simulink model "temp"  (R2015a)
settings: Solver=ode45  StartTime=0.0  StopTime=30.0  RelTol=1e-3
values from neighbouring files (symbols this model uses):
  Kyaw = 4*Kpsi*Km/Izz    (= 8.61428571429)    [Parametros.m]
  ty = 0.0002251891410    (= 0.000225189141)    [Parametros.m]
libraries: simulink x1
settings Model: Creator=DELL  LastModifiedBy=DELL

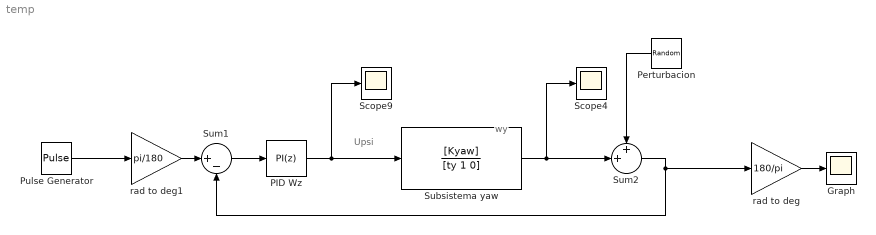
== system temp ==
  note: wy
  note: Upsi
  Graph : Scope
      settings: SaveName=ScopeData3
  PID Wz : simulink/Continuous/PID Controller  Controller=PI  TimeDomain=Discrete-time  SampleTime=0.01  IntegratorMethod=Forward Euler  FilterMethod=Forward Euler  Form=Ideal  UseFilter=on  ControllerParametersSource=internal  P=2.01  I=0.142  D=0.0957187049121133  N=189.58120119176  InitialConditionSource=internal  InitialConditionForIntegrator=0  InitialConditionForFilter=0  ExternalReset=none  LimitOutput=on  UpperSaturationLimit=1  LowerSaturationLimit=-1  LinearizeAsGain=on  AntiWindupMode=back-calculation  Kb=0.1  TrackingMode=off  Kt=1  PParamMin=[]  PParamMax=[]  IParamMin=[]  IParamMax=[]  DParamMin=[]  DParamMax=[]  NParamMin=[]  NParamMax=[]  KbParamMin=[]  KbParamMax=[]  KtParamMin=[]  KtParamMax=[]  POutMin=[]  POutMax=[]  IOutMin=[]  IOutMax=[]  DOutMin=[]  DOutMax=[]  NOutMin=[]  NOutMax=[]  KbOutMin=[]  KbOutMax=[]  KtOutMin=[]  KtOutMax=[]  IntegratorOutMin=[]  IntegratorOutMax=[]  FilterOutMin=[]  FilterOutMax=[]  SumOutMin=[]  SumOutMax=[]  SumI1OutMin=[]  SumI1OutMax=[]  SumI2OutMin=[]  SumI2OutMax=[]  SumI3OutMin=[]  SumI3OutMax=[]  SumDOutMin=[]  SumDOutMax=[]  SaturationOutMin=[]  SaturationOutMax=[]  IntegratorContinuousStateAttributes=''  IntegratorStateMustResolveToSignalObject=off  IntegratorRTWStateStorageClass=Auto  FilterContinuousStateAttributes=''  FilterStateMustResolveToSignalObject=off  FilterRTWStateStorageClass=Auto  DifferentiatorICPrevScaledInput=0  DifferentiatorOutMin=[]  DifferentiatorOutMax=[]
  Perturbacion : RandomNumber  Variance=0.001  Seed=1000  SampleTime=0.01
  Pulse Generator : DiscretePulseGenerator  PulseType=Time based  Amplitude=15  Period=8  PulseWidth=50  PhaseDelay=5
  Scope4 : Scope
      settings: SaveName=ScopeData4
  Scope9 : Scope
      settings: SaveName=ScopeData8
  Subsistema yaw : TransferFcn  Numerator=[Kyaw]  Denominator=[ty 1 0]
  Sum1 : Sum  Inputs=|+-
  Sum2 : Sum  Inputs=++|
  rad to deg : Gain  Gain=180/pi
  rad to deg1 : Gain  Gain=pi/180
  wires:
  Sum1/1 -> PID Wz/1
  Sum2/1 -> rad to deg/1, Sum1/2
  Subsistema yaw/1 -> Scope4/1, Sum2/2
  Pulse Generator/1 -> rad to deg1/1
  PID Wz/1 -> Scope9/1, Subsistema yaw/1
  rad to deg/1 -> Graph/1
  rad to deg1/1 -> Sum1/1
  Perturbacion/1 -> Sum2/1
